simulink model "active_with_narx_and_can"  (R2024a)
settings: Solver=FixedStepAuto  StartTime=0.0  StopTime=40  FixedStep=0.005  RelTol=1e-3
undefined symbols (not defined in the file): A, B, C, canChannel, D, E, H, K1, K2, params, VehicleDataSingle
libraries: neural x41, j1939protocollib x5, vntj1939tllib x1, sldrtlib x1, simulink x1
(part 1 of 3)
settings Model: Creator=lwb  LastModifiedBy=lwb

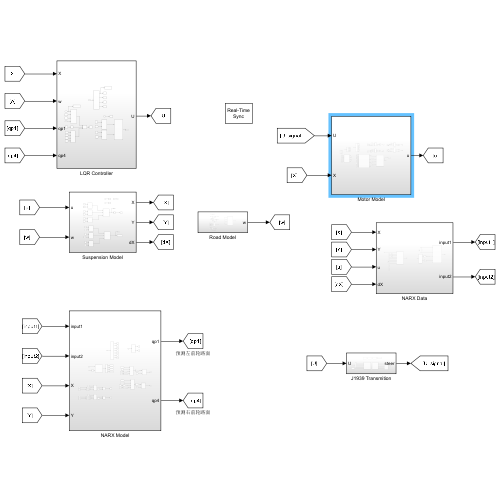
[thumbnail: Simulink's stored preview of the top-level diagram]
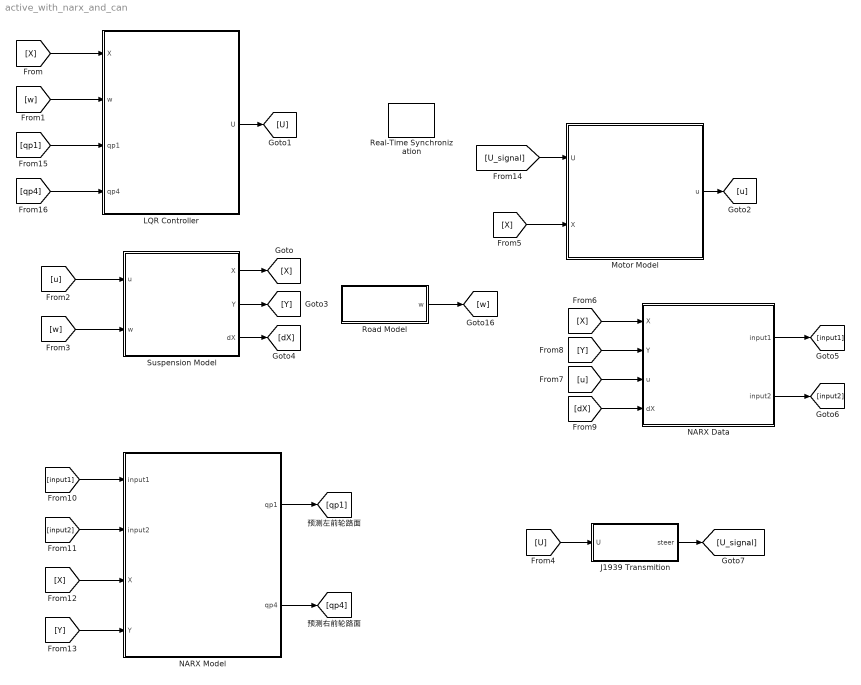
== system active_with_narx_and_can ==
  J1939 Transmition : Subsystem
  LQR Controller : Subsystem
  Motor Model : Subsystem
  NARX Data : Subsystem
  NARX Model : Subsystem
  Real-Time Synchronization : sldrtlib/Real-Time Synchronization  SampleTime=0.1  MaxMissedTicks=10  ShowMissedTicks=off  YieldWhenWaiting=off
  Road Model : Subsystem
  Suspension Model : Subsystem
  wires:
  [X] -> NARX Model/3(X)
  [input1] -> NARX Model/1(input1)
  LQR Controller/1(U) -> [U]
  NARX Data/1(input1) -> [input1]
  [u] -> NARX Data/3(u)
  [input2] -> NARX Model/2(input2)
  Road Model/1(w) -> [w]
  NARX Model/2(qp4) -> [qp4]
  NARX Model/1(qp1) -> [qp1]
  [w] -> LQR Controller/2(w)
  [qp4] -> LQR Controller/4(qp4)
  [u] -> Suspension Model/1(u)
  [Y] -> NARX Model/4(Y)
  [Y] -> NARX Data/2(Y)
  Motor Model/1(u) -> [u]
  NARX Data/2(input2) -> [input2]
  Suspension Model/3(dX) -> [dX]
  [X] -> LQR Controller/1(X)
  Suspension Model/2(Y) -> [Y]
  [dX] -> NARX Data/4(dX)
  [qp1] -> LQR Controller/3(qp1)
  Suspension Model/1(X) -> [X]
  [X] -> Motor Model/2(X)
  [X] -> NARX Data/1(X)
  [w] -> Suspension Model/2(w)
  J1939 Transmition/1(steer) -> [U_signal]
  [U] -> J1939 Transmition/1(U)
  [U_signal] -> Motor Model/1(U)

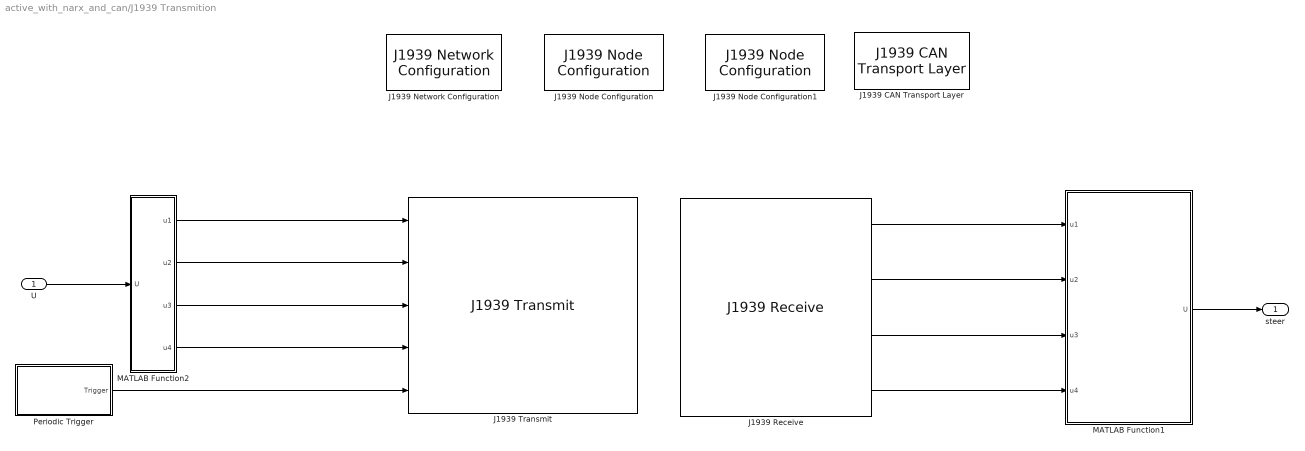
== system active_with_narx_and_can/J1939 Transmition ==
  U : Inport
  " Periodic Trigger" : Subsystem  mask(PeriodicTrigger){repetitionInterval=1}
      mask prompts: repetitionInterval "Repetition Interval (ms):"
      mask help: This block uses the wall-clock time to periodically output a trigger pulse
      mask init:
      | if repetitionInterval < 0
      |  error('xPCTarget:xpcblocks:j1939messagetrigger',...
      |        'Repetition Interval cannot be less than zero');
      | end
      mask Display: disp('Periodic Trigger \n Subsystem');
  J1939 CAN Transport Layer : vntj1939tllib/J1939 CAN Transport Layer  Priority=-2  DeviceMenu=MathWorks Virtual 1 (Channel 1)  ConfigName=Config1  ObjConstructor=canChannel('MathWorks', 'Virtual 1', 1)  Device=MathWorks Virtual 1 (Channel 1)  BusSpeedStr=250000  SampleTime=0.005
  J1939 Network Configuration : j1939protocollib/J1939 Network Configuration  Priority=-3  ConfigName=Config1  DbFile=C:\Users\lwb\Desktop\汽车电子大作业\model\J1939.dbc  PrevDbFile=C:\Users\lwb\Desktop\汽车电子大作业\model\J1939.dbc  enableAC=on
  J1939 Node Configuration : j1939protocollib/J1939 Node Configuration  Priority=-2  ConfigName=Config1  NodeID=Node1  NodeName=Node1  PrevNodeID=Custom  PrevConfig=Config  AllowAAC=off  NodeAddress=30  IndustryGroup=0  VehicleSystem=0  VehicleSystemInstance=0  FunctionID=22  FunctionInstance=0  ECUInstance=0  ManufacturerCode=0  IDNumber=0  SampleTime=0.005  OutputAddress=off  OutputACStatus=off
  J1939 Node Configuration1 : j1939protocollib/J1939 Node Configuration  Priority=-2  ConfigName=Config1  NodeID=Node2  NodeName=Node2  PrevNodeID=Custom  PrevConfig=Config  AllowAAC=off  NodeAddress=50  IndustryGroup=0  VehicleSystem=0  VehicleSystemInstance=0  FunctionID=8  FunctionInstance=0  ECUInstance=0  ManufacturerCode=0  IDNumber=0  SampleTime=0.005  OutputAddress=off  OutputACStatus=off
  J1939 Receive : j1939protocollib/J1939 Receive  Priority=-1  ConfigName=Config1  NodeName=Node2  PGList=VehicleDataSingle(40192)  PGName=VehicleDataSingle  MsgLength=8  SignalInfo=VehicleSignal1$0$16$1$1$1$0$1$0$-Inf$Inf$$0$#VehicleSignal2$16$16$1$1$1$0$1$0$-Inf$Inf$$0$#VehicleSignal3$32$16$1$1$1$0$1$0$-Inf$Inf$$0$#VehicleSignal4$48$16$1$1$1$0$1$0$-Inf$Inf$$0$#  NSignals=4  StartBits=str2num('[double(0);double(16);double(32);double(48)]')  SignalSizes=str2num('[double(16),double(16),double(16),double(16)]')  ByteOrders=str2num('[int32(1);int32(1);int32(1);int32(1)]')  DataTypes=str2num('[int32(1);int32(1);int32(1);int32(1)]')  MultiplexTypes=str2num('[int32(1);int32(1);int32(1);int32(1)]')  MultiplexValues=str2num('[double(0);double(0);double(0);double(0)]')  Factors=str2num('[double(1);double(1);double(1);double(1)]')  Offsets=str2num('[double(0);double(0);double(0);double(0)]')  Minimums=str2num('[double(-Inf);double(-Inf);double(-Inf);double(-Inf)]')  Maximums=str2num('[double(Inf);double(Inf);double(Inf);double(Inf)]')  Units=0  SPN=str2num('[double(0);double(0);double(0);double(0)]')  Comment=0  SrcAddrFilter=Allow all  SrcAddress=255  DestAddrFilter=1  outputNew=off  SampleTime=0.005  ApplyMinMax=off
  J1939 Transmit : j1939protocollib/J1939 Transmit  Priority=-1  ConfigName=Config1  NodeName=Node1  PGList=VehicleDataSingle(40192)  PGName=VehicleDataSingle  MsgLength=8  SignalInfo=VehicleSignal1$0$16$1$1$1$0$1$0$-Inf$Inf$$0$#VehicleSignal2$16$16$1$1$1$0$1$0$-Inf$Inf$$0$#VehicleSignal3$32$16$1$1$1$0$1$0$-Inf$Inf$$0$#VehicleSignal4$48$16$1$1$1$0$1$0$-Inf$Inf$$0$#  NSignals=4  StartBits=str2num('[double(0);double(16);double(32);double(48)]')  SignalSizes=str2num('[double(16),double(16),double(16),double(16)]')  ByteOrders=str2num('[int32(1);int32(1);int32(1);int32(1)]')  DataTypes=str2num('[int32(1);int32(1);int32(1);int32(1)]')  MultiplexTypes=str2num('[int32(1);int32(1);int32(1);int32(1)]')  MultiplexValues=str2num('[double(0);double(0);double(0);double(0)]')  Factors=str2num('[double(1);double(1);double(1);double(1)]')  Offsets=str2num('[double(0);double(0);double(0);double(0)]')  Minimums=str2num('[double(-Inf);double(-Inf);double(-Inf);double(-Inf)]')  Maximums=str2num('[double(Inf);double(Inf);double(Inf);double(Inf)]')  Units=0  SPN=str2num('[double(0);double(0);double(0);double(0)]')  Comment=0  PGPriority=6  DestAddrID=Node2  DestAddrName=50  TransmitPeriodically=on  MessagePeriod=0  SampleTime=-1  ApplyMinMax=off
  MATLAB Function1 : MATLAB Function  TreatAsAtomicUnit=on
  MATLAB Function2 : MATLAB Function  TreatAsAtomicUnit=on
  steer : Outport
  wires:
  U/1 -> MATLAB Function2/1(U)
  MATLAB Function1/1(U) -> steer/1
  " Periodic Trigger"/1(Trigger) -> J1939 Transmit/5
  MATLAB Function2/1(u1) -> J1939 Transmit/1
  MATLAB Function2/2(u2) -> J1939 Transmit/2
  MATLAB Function2/3(u3) -> J1939 Transmit/3
  MATLAB Function2/4(u4) -> J1939 Transmit/4
  J1939 Receive/1 -> MATLAB Function1/1(u1)
  J1939 Receive/2 -> MATLAB Function1/2(u2)
  J1939 Receive/3 -> MATLAB Function1/3(u3)
  J1939 Receive/4 -> MATLAB Function1/4(u4)

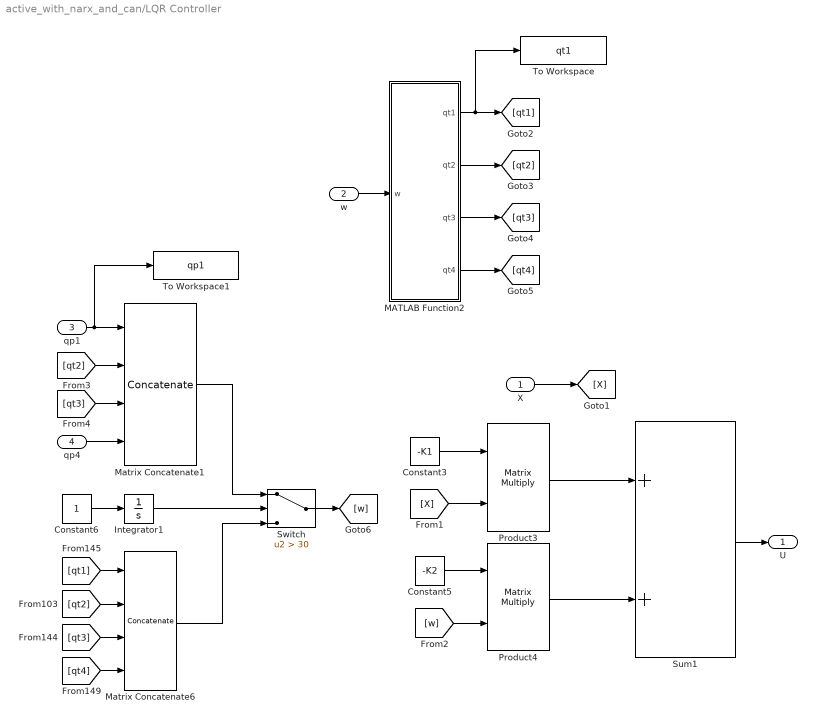
== system active_with_narx_and_can/LQR Controller ==
  X : Inport
  w : Inport  Port=2
  qp1 : Inport  Port=3
  qp4 : Inport  Port=4
  Constant3 : Constant  Value=-K1  VectorParams1D=off
  Constant5 : Constant  Value=-K2  VectorParams1D=off
  Constant6 : Constant
  Integrator1 : Integrator
  MATLAB Function2 : MATLAB Function  TreatAsAtomicUnit=on
  Matrix Concatenate1 : Concatenate  NumInputs=4  Mode=Multidimensional array
  Matrix Concatenate6 : Concatenate  NumInputs=4  Mode=Multidimensional array
  Product3 : Product  Multiplication=Matrix(*)
  Product4 : Product  Multiplication=Matrix(*)
  Sum1 : Sum
  Switch : Switch  Criteria=u2 > Threshold  Threshold=30  SaturateOnIntegerOverflow=off  InputSameDT=off
  To Workspace : ToWorkspace  VariableName=qt1  SaveFormat=Timeseries  SampleTime=-1
  To Workspace1 : ToWorkspace  VariableName=qp1  SaveFormat=Timeseries  SampleTime=-1
  U : Outport
  wires:
  [X] -> Product3/2
  Constant5/1 -> Product4/1
  Constant3/1 -> Product3/1
  Sum1/1 -> U/1
  Product3/1 -> Sum1/1
  Product4/1 -> Sum1/2
  [w] -> Product4/2
  X/1 -> [X]
  [qt2] -> Matrix Concatenate6/2
  [qt4] -> Matrix Concatenate6/4
  [qt3] -> Matrix Concatenate6/3
  Constant6/1 -> Integrator1/1
  [qt1] -> Matrix Concatenate6/1
  Integrator1/1 -> Switch/2
  w/1 -> MATLAB Function2/1(w)
  Switch/1 -> [w]
  qp1/1 -> To Workspace1/1, Matrix Concatenate1/1
  [qt2] -> Matrix Concatenate1/2
  qp4/1 -> Matrix Concatenate1/4
  [qt3] -> Matrix Concatenate1/3
  Matrix Concatenate1/1 -> Switch/1
  Matrix Concatenate6/1 -> Switch/3
  MATLAB Function2/3(qt3) -> [qt3]
  MATLAB Function2/2(qt2) -> [qt2]
  MATLAB Function2/4(qt4) -> [qt4]
  MATLAB Function2/1(qt1) -> To Workspace/1, [qt1]

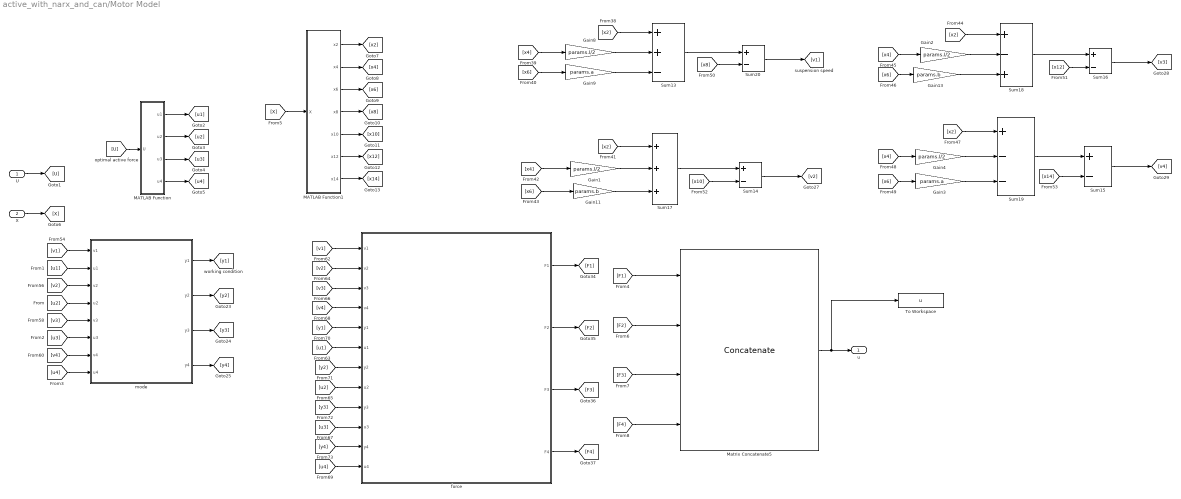
== system active_with_narx_and_can/Motor Model ==
  U : Inport
  X : Inport  Port=2
  Gain{1..2,4,8} (4 alike) : Gain  Gain=params.l/2
  Gain11 : Gain  Gain=params.b
  Gain13 : Gain  Gain=params.b
  Gain3 : Gain  Gain=params.a
  Gain9 : Gain  Gain=params.a
  MATLAB Function : MATLAB Function  TreatAsAtomicUnit=on
  MATLAB Function1 : MATLAB Function  TreatAsAtomicUnit=on
  Matrix Concatenate5 : Concatenate  NumInputs=4  Mode=Multidimensional array
  Sum13 : Sum  Inputs=++-
  Sum{14..16,20} (4 alike) : Sum  Inputs=+-
  Sum17 : Sum  Inputs=+++
  Sum18 : Sum  Inputs=+-+
  Sum19 : Sum  Inputs=+--
  To Workspace : ToWorkspace  VariableName=u  SaveFormat=Timeseries  SampleTime=-1
  force : Subsystem
  mode : Subsystem
  u : Outport
  wires:
  [y4] -> force/11(y4)
  [u1] -> force/6(u1)
  force/1(F1) -> [F1]
  force/2(F2) -> [F2]
  [v2] -> force/2(v2)
  mode/1(y1) -> [y1]
  [v3] -> force/3(v3)
  [u4] -> mode/8(u4)
  [u3] -> mode/6(u3)
  force/4(F4) -> [F4]
  [v4] -> force/4(v4)
  [y2] -> force/7(y2)
  [v3] -> mode/5(v3)
  mode/2(y2) -> [y2]
  [v4] -> mode/7(v4)
  [u4] -> force/12(u4)
  mode/4(y4) -> [y4]
  [u3] -> force/10(u3)
  mode/3(y3) -> [y3]
  [v2] -> mode/3(v2)
  [u2] -> force/8(u2)
  [v1] -> force/1(v1)
  [v1] -> mode/1(v1)
  [u2] -> mode/4(u2)
  [y3] -> force/9(y3)
  [u1] -> mode/2(u1)
  force/3(F3) -> [F3]
  [y1] -> force/5(y1)
  Sum19/1 -> Sum15/1
  [x14] -> Sum15/2
  Sum16/1 -> [v3]
  [x6] -> Gain13/1
  Gain8/1 -> Sum13/2
  [x2] -> Sum13/1
  Gain1/1 -> Sum17/2
  Sum20/1 -> [v1]
  [x2] -> Sum19/1
  [x4] -> Gain4/1
  [x6] -> Gain9/1
  [x2] -> Sum18/1
  Sum18/1 -> Sum16/1
  Gain9/1 -> Sum13/3
  Sum13/1 -> Sum20/1
  [x12] -> Sum16/2
  Sum15/1 -> [v4]
  Gain3/1 -> Sum19/3
  Gain2/1 -> Sum18/2
  [x4] -> Gain2/1
  [x4] -> Gain1/1
  Gain13/1 -> Sum18/3
  [x6] -> Gain11/1
  Sum17/1 -> Sum14/1
  Gain11/1 -> Sum17/3
  Gain4/1 -> Sum19/2
  [x10] -> Sum14/2
  [x2] -> Sum17/1
  [x4] -> Gain8/1
  Sum14/1 -> [v2]
  [x6] -> Gain3/1
  [x8] -> Sum20/2
  U/1 -> [U]
  [U] -> MATLAB Function/1(U)
  MATLAB Function/2(u2) -> [u2]
  MATLAB Function/3(u3) -> [u3]
  MATLAB Function/4(u4) -> [u4]
  MATLAB Function/1(u1) -> [u1]
  X/1 -> [X]
  [X] -> MATLAB Function1/1(X)
  MATLAB Function1/1(x2) -> [x2]
  MATLAB Function1/2(x4) -> [x4]
  MATLAB Function1/3(x6) -> [x6]
  MATLAB Function1/4(x8) -> [x8]
  MATLAB Function1/5(x10) -> [x10]
  MATLAB Function1/6(x12) -> [x12]
  MATLAB Function1/7(x14) -> [x14]
  [F1] -> Matrix Concatenate5/1
  [F3] -> Matrix Concatenate5/3
  [F4] -> Matrix Concatenate5/4
  [F2] -> Matrix Concatenate5/2
  Matrix Concatenate5/1 -> To Workspace/1, u/1

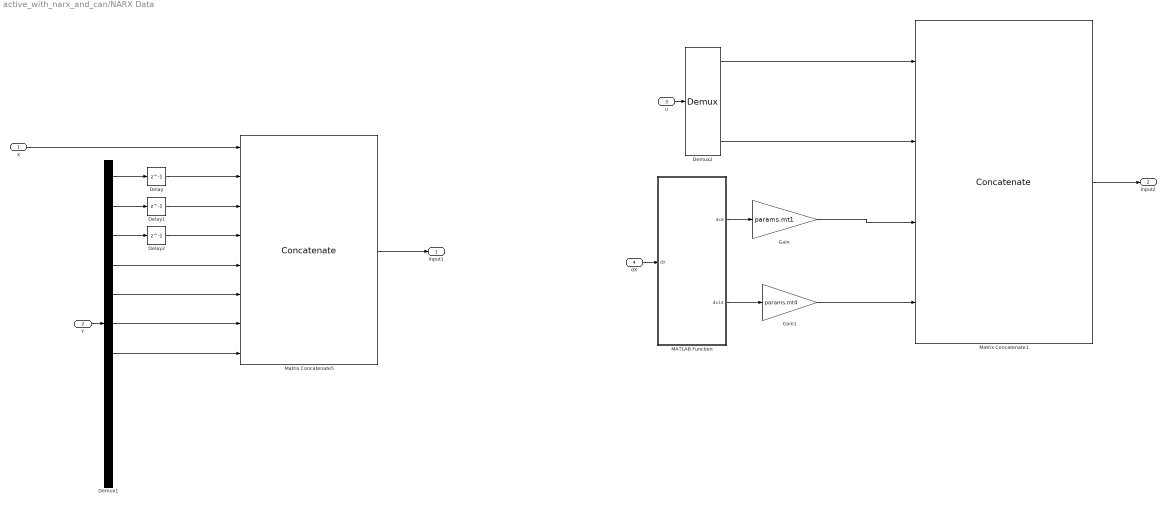
== system active_with_narx_and_can/NARX Data ==
  X : Inport
  Y : Inport  Port=2
  u : Inport  Port=3
  dX : Inport  Port=4
  Delay : Delay  DelayLength=1
  Delay1 : Delay  DelayLength=1
  Delay2 : Delay  DelayLength=1
  Demux1 : Demux  Outputs=11
  Demux2 : Demux
  Gain : Gain  Gain=params.mt1
  Gain1 : Gain  Gain=params.mt4
  MATLAB Function : MATLAB Function  TreatAsAtomicUnit=on
  Matrix Concatenate1 : Concatenate  NumInputs=4  Mode=Multidimensional array
  Matrix Concatenate5 : Concatenate  NumInputs=8  Mode=Multidimensional array
  input1 : Outport
  input2 : Outport  Port=2
  wires:
  Y/1 -> Demux1/1
  Demux1/1 -> Delay/1
  Demux1/2 -> Delay1/1
  Demux1/3 -> Delay2/1
  u/1 -> Demux2/1
  Demux2/1 -> Matrix Concatenate1/1
  Demux2/4 -> Matrix Concatenate1/2
  dX/1 -> MATLAB Function/1(dX)
  MATLAB Function/1(dx8) -> Gain/1
  MATLAB Function/2(dx14) -> Gain1/1
  Gain/1 -> Matrix Concatenate1/3
  Gain1/1 -> Matrix Concatenate1/4
  X/1 -> Matrix Concatenate5/1
  Delay/1 -> Matrix Concatenate5/2
  Delay1/1 -> Matrix Concatenate5/3
  Delay2/1 -> Matrix Concatenate5/4
  Demux1/4 -> Matrix Concatenate5/5
  Demux1/5 -> Matrix Concatenate5/6
  Demux1/6 -> Matrix Concatenate5/7
  Demux1/7 -> Matrix Concatenate5/8
  Matrix Concatenate5/1 -> input1/1
  Matrix Concatenate1/1 -> input2/1

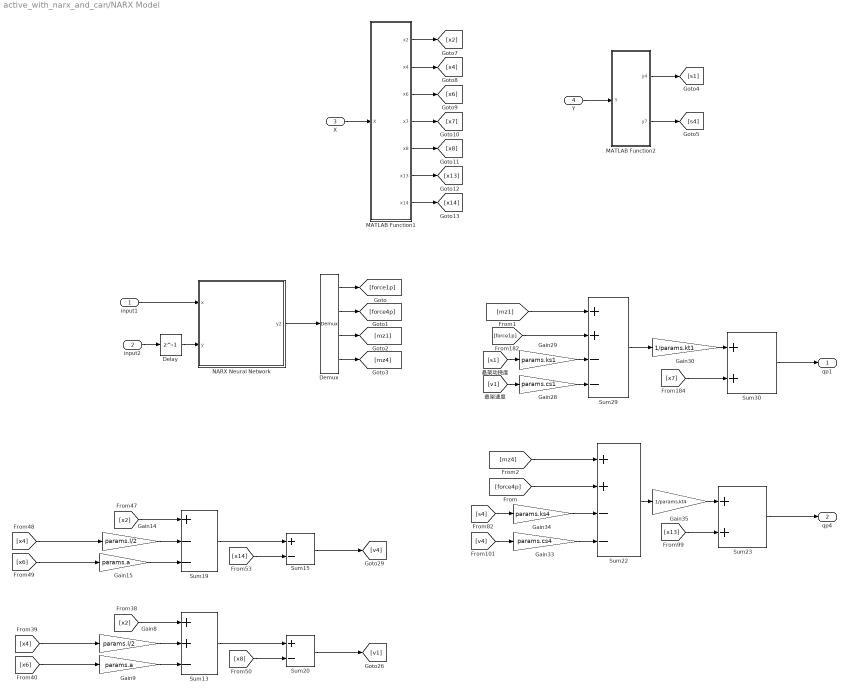
== system active_with_narx_and_can/NARX Model ==
  input1 : Inport
  input2 : Inport  Port=2
  X : Inport  Port=3
  Y : Inport  Port=4
  Delay : Delay  DelayLength=1
  Demux : Demux
  Gain14 : Gain  Gain=params.l/2
  Gain15 : Gain  Gain=params.a
  Gain28 : Gain  Gain=params.cs1
  Gain29 : Gain  Gain=params.ks1
  Gain30 : Gain  Gain=1/params.kt1
  Gain33 : Gain  Gain=params.cs4
  Gain34 : Gain  Gain=params.ks4
  Gain35 : Gain  Gain=1/params.kt4
  Gain8 : Gain  Gain=params.l/2
  Gain9 : Gain  Gain=params.a
  MATLAB Function1 : MATLAB Function  TreatAsAtomicUnit=on
  MATLAB Function2 : MATLAB Function  TreatAsAtomicUnit=on
  NARX Neural Network : Subsystem  mask{pi_input_1_delayed_1=[0;0;0;0;0;0;0;0;0;0;0;0;0;0;0;0;0;0;0;0;0], pi_input_1_delayed_2=[0;0;0;0;0;0;0;0;0;0;0;0;0;0;0;0;0;0;0;0;0], pi_input_2_delayed_1=[0;0;0;0], pi_input_2_delayed_2=[0;0;0;0]}
      mask prompts: pi_input_1_delayed_1 "Preprocessed initial input 1 state at timestep 0."; pi_input_1_delayed_2 "Preprocessed initial input 1 state at timestep -1."; pi_input_2_delayed_1 "Preprocessed initial input 2 state at timestep 0."; pi_input_2_delayed_2 "Preprocessed initial input 2 state at timestep -1."
      mask help: NARX Neural Network
      mask Display: e = 0.06;c1 = [120 150 230]/255;c2 = ([120 150 230]+0)/383;c3 = ([120 150 230]+128)/383;patch([0 1 1 0],[0 0 1 1],c1);patch([0 1 1 1-e 1-e 0+e],[0 0 1 1-e 0+e 0+e],c2);patch([0 0 1 1-e 0+e 0+e],[0 1 1 1-e 1-e 0+e],c3);plot([0 1 1 0 0],[0 0 1 1 0]);fprintf('NNET');port_label('input',1,' x');port_label('input',2,' y');port_label('output',1,'y2 ');
  Sum13 : Sum  Inputs=++-
  Sum15 : Sum  Inputs=+-
  Sum19 : Sum  Inputs=+--
  Sum20 : Sum  Inputs=+-
  Sum22 : Sum  Inputs=++--
  Sum23 : Sum
  Sum29 : Sum  Inputs=++--
  Sum30 : Sum
  qp1 : Outport
  qp4 : Outport  Port=2
  wires:
  Delay/1 -> NARX Neural Network/2(y)
  input2/1 -> Delay/1
  input1/1 -> NARX Neural Network/1(x)
  Gain30/1 -> Sum30/1
  Sum30/1 -> qp1/1
  Gain29/1 -> Sum29/3
  Gain33/1 -> Sum22/4
  [v1] -> Gain28/1
  [x13] -> Sum23/2
  [force4p] -> Sum22/2
  Gain35/1 -> Sum23/1
  [s1] -> Gain29/1
  Sum29/1 -> Gain30/1
  Sum22/1 -> Gain35/1
  Gain34/1 -> Sum22/3
  [s4] -> Gain34/1
  [force1p] -> Sum29/2
  Sum23/1 -> qp4/1
  [v4] -> Gain33/1
  [mz1] -> Sum29/1
  [mz4] -> Sum22/1
  [x7] -> Sum30/2
  Gain28/1 -> Sum29/4
  NARX Neural Network/1(y2) -> Demux/1
  Demux/1 -> [force1p]
  Demux/2 -> [force4p]
  Demux/3 -> [mz1]
  Demux/4 -> [mz4]
  [x2] -> Sum13/1
  [x4] -> Gain14/1
  [x8] -> Sum20/2
  Sum19/1 -> Sum15/1
  [x14] -> Sum15/2
  Sum13/1 -> Sum20/1
  Sum20/1 -> [v1]
  Gain14/1 -> Sum19/2
  [x6] -> Gain9/1
  Gain9/1 -> Sum13/3
  [x4] -> Gain8/1
  Sum15/1 -> [v4]
  Gain8/1 -> Sum13/2
  [x2] -> Sum19/1
  [x6] -> Gain15/1
  Gain15/1 -> Sum19/3
  MATLAB Function1/6(x13) -> [x13]
  MATLAB Function1/1(x2) -> [x2]
  MATLAB Function1/2(x4) -> [x4]
  MATLAB Function1/3(x6) -> [x6]
  X/1 -> MATLAB Function1/1(X)
  MATLAB Function1/7(x14) -> [x14]
  MATLAB Function1/4(x7) -> [x7]
  MATLAB Function1/5(x8) -> [x8]
  Y/1 -> MATLAB Function2/1(Y)
  MATLAB Function2/1(y4) -> [s1]
  MATLAB Function2/2(y7) -> [s4]

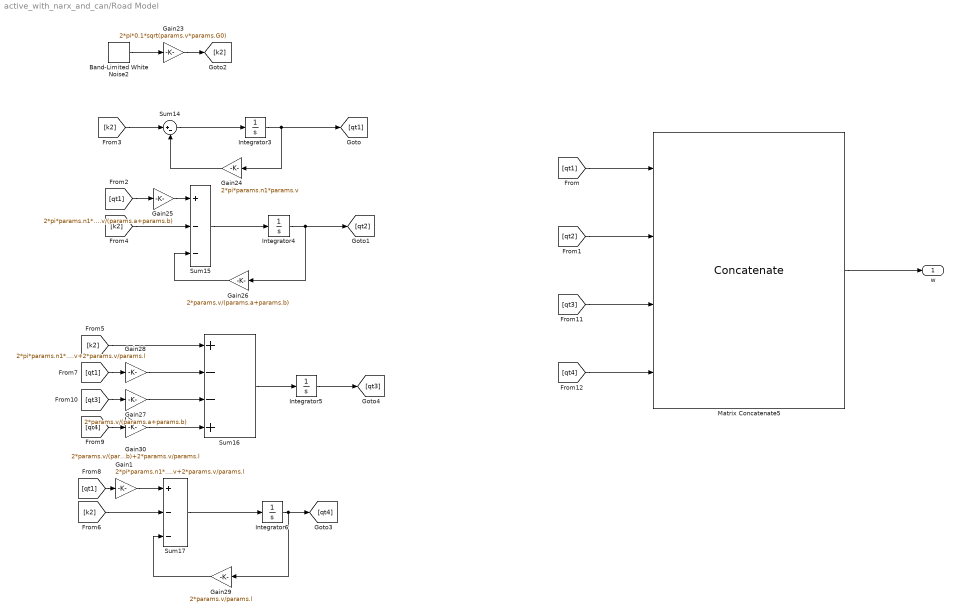
== system active_with_narx_and_can/Road Model ==
  Band-Limited White Noise2 : simulink/Sources/Band-Limited White Noise  Cov=[0.5]  Ts=1/10/params.v  seed=[23341]
  Gain1 : Gain  Gain=2*pi*params.n1*params.v+2*params.v/params.l
  Gain23 : Gain  Gain=2*pi*0.1*sqrt(params.v*params.G0)
  Gain24 : Gain  Gain=2*pi*params.n1*params.v
  Gain25 : Gain  Gain=2*pi*params.n1*params.v+2*params.v/(params.a+params.b)
  Gain26 : Gain  Gain=2*params.v/(params.a+params.b)
  Gain27 : Gain  Gain=2*params.v/(params.a+params.b)
  Gain28 : Gain  Gain=2*pi*params.n1*params.v+2*params.v/params.l
  Gain29 : Gain  Gain=2*params.v/params.l
  Gain30 : Gain  Gain=2*params.v/(params.a+params.b)+2*params.v/params.l
  Integrator{3..6} (4 alike) : Integrator
  Matrix Concatenate5 : Concatenate  NumInputs=4  Mode=Multidimensional array
  Sum14 : Sum  Inputs=|+-
  Sum15 : Sum  Inputs=+--
  Sum16 : Sum  Inputs=+--+
  Sum17 : Sum  Inputs=+--
  w : Outport
  wires:
  Gain25/1 -> Sum15/1
  Gain27/1 -> Sum16/3
  Gain26/1 -> Sum15/3
  Gain24/1 -> Sum14/2
  Integrator5/1 -> [qt3]
  Integrator3/1 -> Gain24/1, [qt1]
  Matrix Concatenate5/1 -> w/1
  Sum14/1 -> Integrator3/1
  Integrator4/1 -> Gain26/1, [qt2]
  Integrator6/1 -> Gain29/1, [qt4]
  Gain28/1 -> Sum16/2
  Gain29/1 -> Sum17/3
  Sum16/1 -> Integrator5/1
  Sum15/1 -> Integrator4/1
  Gain30/1 -> Sum16/4
  Sum17/1 -> Integrator6/1
  [k2] -> Sum14/1
  Band-Limited White Noise2/1 -> Gain23/1
  Gain23/1 -> [k2]
  [k2] -> Sum15/2
  [k2] -> Sum16/1
  [k2] -> Sum17/2
  [qt1] -> Gain25/1
  [qt1] -> Gain28/1
  [qt1] -> Gain1/1
  Gain1/1 -> Sum17/1
  [qt3] -> Gain27/1
  [qt4] -> Gain30/1
  [qt3] -> Matrix Concatenate5/3
  [qt4] -> Matrix Concatenate5/4
  [qt1] -> Matrix Concatenate5/1
  [qt2] -> Matrix Concatenate5/2

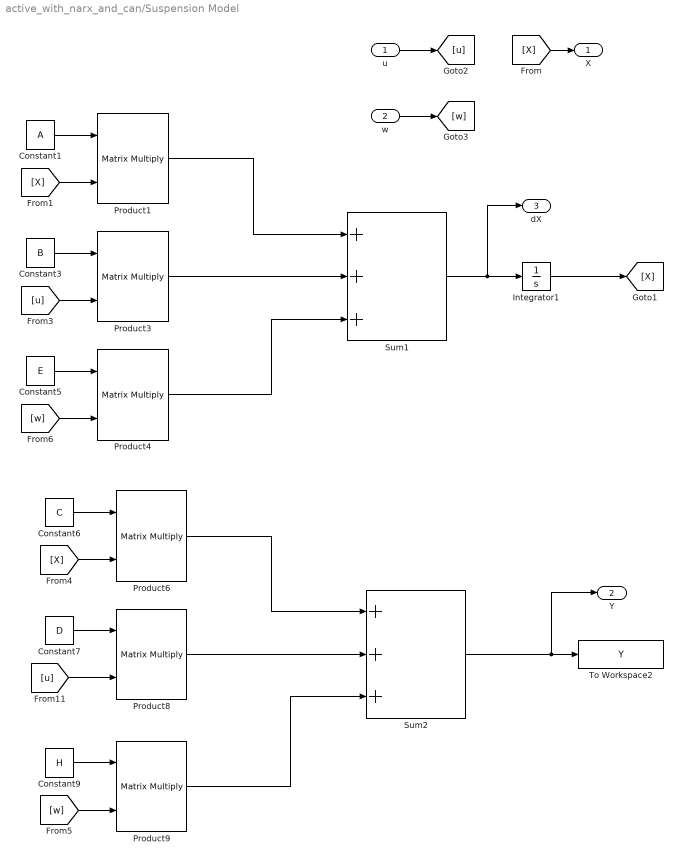
== system active_with_narx_and_can/Suspension Model ==
  u : Inport
  w : Inport  Port=2
  Constant1 : Constant  Value=A  VectorParams1D=off
  Constant3 : Constant  Value=B  VectorParams1D=off
  Constant5 : Constant  Value=E  VectorParams1D=off
  Constant6 : Constant  Value=C  VectorParams1D=off
  Constant7 : Constant  Value=D  VectorParams1D=off
  Constant9 : Constant  Value=H  VectorParams1D=off
  Integrator1 : Integrator
  Product{1,3..4,6,8..9} (6 alike) : Product  Multiplication=Matrix(*)
  Sum1 : Sum  Inputs=+++
  Sum2 : Sum  Inputs=+++
  To Workspace2 : ToWorkspace  VariableName=Y  SaveFormat=Timeseries  SampleTime=-1
  X : Outport
  Y : Outport  Port=2
  dX : Outport  Port=3
  wires:
  Constant3/1 -> Product3/1
  [u] -> Product8/2
  Product4/1 -> Sum1/3
  [u] -> Product3/2
  Product1/1 -> Sum1/1
  Constant1/1 -> Product1/1
  Product6/1 -> Sum2/1
  Sum1/1 -> dX/1, Integrator1/1
  Product9/1 -> Sum2/3
  [X] -> Product1/2
  Product8/1 -> Sum2/2
  Constant7/1 -> Product8/1
  [w] -> Product9/2
  Constant9/1 -> Product9/1
  Constant6/1 -> Product6/1
  Sum2/1 -> Y/1, To Workspace2/1
  Product3/1 -> Sum1/2
  [X] -> Product6/2
  [w] -> Product4/2
  Constant5/1 -> Product4/1
  u/1 -> [u]
  w/1 -> [w]
  Integrator1/1 -> [X]
  [X] -> X/1

== system active_with_narx_and_can/J1939 Transmition/ Periodic Trigger ==
  Relational Operator : RelationalOperator  OutDataTypeStr=boolean  InputSameDT=off
  Repetition Interval : Constant  Value=repetitionInterval
  Timer : Subsystem
  Unit Delay : UnitDelay  InitialCondition=1  SampleTime=-1  HasFrameUpgradeWarning=on
  Trigger : Outport  OutputWhenDisabled=reset  InitialOutput=0  VectorParamsAs1DForOutWhenUnconnected=off
  wires:
  Timer/1(Timer Value (ms)) -> Relational Operator/1
  Repetition Interval/1 -> Relational Operator/2
  Unit Delay/1 -> Timer/1(Reset)
  Relational Operator/1 -> Trigger/1, Unit Delay/1  "Trigger Pulse"

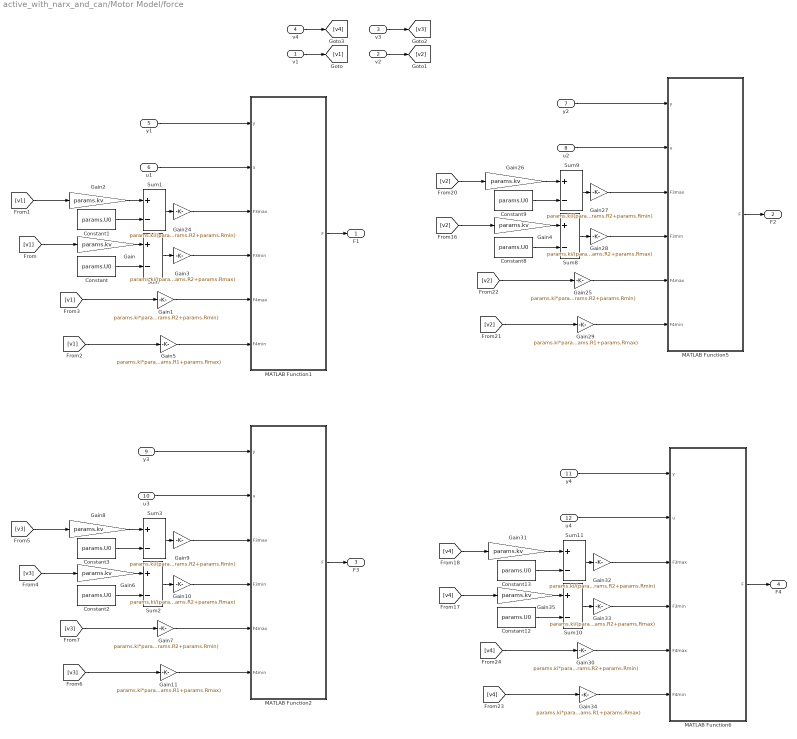
== system active_with_narx_and_can/Motor Model/force ==
  v1 : Inport
  v2 : Inport  Port=2
  v3 : Inport  Port=3
  v4 : Inport  Port=4
  y1 : Inport  Port=5
  u1 : Inport  Port=6
  y2 : Inport  Port=7
  u2 : Inport  Port=8
  y3 : Inport  Port=9
  u3 : Inport  Port=10
  y4 : Inport  Port=11
  u4 : Inport  Port=12
  Constant{,1..3,8..9,12..13} (8 alike) : Constant  Value=params.U0
  Gain{,2,4,6,8,26,31,35} (8 alike) : Gain  Gain=params.kv
  Gain{1,7,25,30} (4 alike) : Gain  Gain=params.ki*params.kv/(params.R2+params.Rmin)
  Gain{3,10,28,33} (4 alike) : Gain  Gain=params.ki/(params.R1+params.R2+params.Rmax)
  Gain{5,11,29,34} (4 alike) : Gain  Gain=params.ki*params.kv/(params.R1+params.Rmax)
  Gain{9,24,27,32} (4 alike) : Gain  Gain=params.ki/(params.R1+params.R2+params.Rmin)
  MATLAB Function1 : MATLAB Function  TreatAsAtomicUnit=on
  MATLAB Function2 : MATLAB Function  TreatAsAtomicUnit=on
  MATLAB Function5 : MATLAB Function  TreatAsAtomicUnit=on
  MATLAB Function6 : MATLAB Function  TreatAsAtomicUnit=on
  Sum{,1..3,8..11} (8 alike) : Sum  Inputs=+-
  F1 : Outport
  F2 : Outport  Port=2
  F3 : Outport  Port=3
  F4 : Outport  Port=4
  wires:
  v4/1 -> [v4]
  Gain3/1 -> MATLAB Function1/4(F3min)
  Gain1/1 -> MATLAB Function1/5(F4max)
  v3/1 -> [v3]
  v2/1 -> [v2]
  [v1] -> Gain1/1
  Gain5/1 -> MATLAB Function1/6(F4min)
  Gain24/1 -> MATLAB Function1/3(F3max)
  [v1] -> Gain/1
  v1/1 -> [v1]
  Constant1/1 -> Sum1/2
  Sum1/1 -> Gain24/1
  Sum/1 -> Gain3/1
  Constant/1 -> Sum/2
  Gain/1 -> Sum/1
  y1/1 -> MATLAB Function1/1(y)
  u1/1 -> MATLAB Function1/2(u)
  [v1] -> Gain2/1
  Gain2/1 -> Sum1/1
  [v1] -> Gain5/1
  MATLAB Function1/1(F) -> F1/1
  MATLAB Function5/1(F) -> F2/1
  [v2] -> Gain29/1
  Gain26/1 -> Sum9/1
  [v2] -> Gain26/1
  u2/1 -> MATLAB Function5/2(u)
  y2/1 -> MATLAB Function5/1(y)
  Gain4/1 -> Sum8/1
  Constant8/1 -> Sum8/2
  Sum8/1 -> Gain28/1
  Sum9/1 -> Gain27/1
  Constant9/1 -> Sum9/2
  [v2] -> Gain4/1
  Gain27/1 -> MATLAB Function5/3(F3max)
  Gain29/1 -> MATLAB Function5/6(F4min)
  [v2] -> Gain25/1
  Gain25/1 -> MATLAB Function5/5(F4max)
  Gain28/1 -> MATLAB Function5/4(F3min)
  MATLAB Function2/1(F) -> F3/1
  [v3] -> Gain11/1
  Gain8/1 -> Sum3/1
  [v3] -> Gain8/1
  u3/1 -> MATLAB Function2/2(u)
  y3/1 -> MATLAB Function2/1(y)
  Gain6/1 -> Sum2/1
  Constant2/1 -> Sum2/2
  Sum2/1 -> Gain10/1
  Sum3/1 -> Gain9/1
  Constant3/1 -> Sum3/2
  [v3] -> Gain6/1
  Gain9/1 -> MATLAB Function2/3(F3max)
  Gain11/1 -> MATLAB Function2/6(F4min)
  [v3] -> Gain7/1
  Gain7/1 -> MATLAB Function2/5(F4max)
  Gain10/1 -> MATLAB Function2/4(F3min)
  Gain33/1 -> MATLAB Function6/4(F3min)
  Gain30/1 -> MATLAB Function6/5(F4max)
  [v4] -> Gain30/1
  Gain34/1 -> MATLAB Function6/6(F4min)
  Gain32/1 -> MATLAB Function6/3(F3max)
  [v4] -> Gain35/1
  Constant13/1 -> Sum11/2
  Sum11/1 -> Gain32/1
  Sum10/1 -> Gain33/1
  Constant12/1 -> Sum10/2
  Gain35/1 -> Sum10/1
  y4/1 -> MATLAB Function6/1(y)
  u4/1 -> MATLAB Function6/2(u)
  [v4] -> Gain31/1
  Gain31/1 -> Sum11/1
  [v4] -> Gain34/1
  MATLAB Function6/1(F) -> F4/1

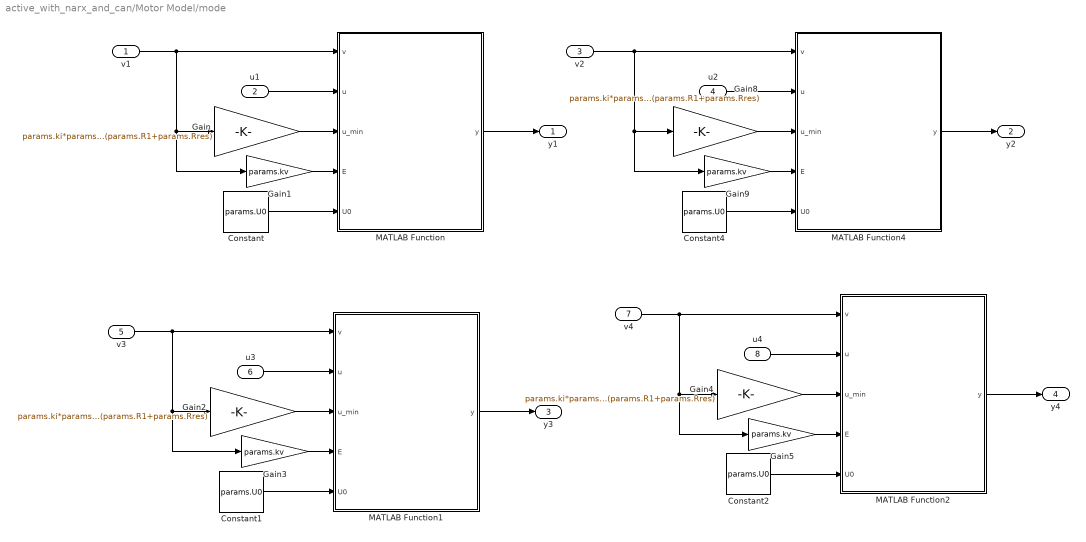
== system active_with_narx_and_can/Motor Model/mode ==
  v1 : Inport
  u1 : Inport  Port=2
  v2 : Inport  Port=3
  u2 : Inport  Port=4
  v3 : Inport  Port=5
  u3 : Inport  Port=6
  v4 : Inport  Port=7
  u4 : Inport  Port=8
  Constant{,1..2,4} (4 alike) : Constant  Value=params.U0
  Gain{,2,4,8} (4 alike) : Gain  Gain=params.ki*params.kv/(params.R1+params.Rres)
  Gain{1,3,5,9} (4 alike) : Gain  Gain=params.kv
  MATLAB Function : MATLAB Function  TreatAsAtomicUnit=on
  MATLAB Function1 : MATLAB Function  TreatAsAtomicUnit=on
  MATLAB Function2 : MATLAB Function  TreatAsAtomicUnit=on
  MATLAB Function4 : MATLAB Function  TreatAsAtomicUnit=on
  y1 : Outport
  y2 : Outport  Port=2
  y3 : Outport  Port=3
  y4 : Outport  Port=4
  wires:
  v1/1 -> MATLAB Function/1(v), Gain1/1, Gain/1
  u1/1 -> MATLAB Function/2(u)
  Gain/1 -> MATLAB Function/3(u_min)
  Gain1/1 -> MATLAB Function/4(E)
  Constant/1 -> MATLAB Function/5(U0)
  MATLAB Function/1(y) -> y1/1
  MATLAB Function4/1(y) -> y2/1
  Constant4/1 -> MATLAB Function4/5(U0)
  Gain9/1 -> MATLAB Function4/4(E)
  Gain8/1 -> MATLAB Function4/3(u_min)
  u2/1 -> MATLAB Function4/2(u)
  v2/1 -> Gain8/1, Gain9/1, MATLAB Function4/1(v)
  MATLAB Function1/1(y) -> y3/1
  Constant1/1 -> MATLAB Function1/5(U0)
  Gain3/1 -> MATLAB Function1/4(E)
  Gain2/1 -> MATLAB Function1/3(u_min)
  u3/1 -> MATLAB Function1/2(u)
  v3/1 -> Gain2/1, Gain3/1, MATLAB Function1/1(v)
  v4/1 -> MATLAB Function2/1(v), Gain5/1, Gain4/1
  u4/1 -> MATLAB Function2/2(u)
  Gain4/1 -> MATLAB Function2/3(u_min)
  Gain5/1 -> MATLAB Function2/4(E)
  Constant2/1 -> MATLAB Function2/5(U0)
  MATLAB Function2/1(y) -> y4/1

== system active_with_narx_and_can/NARX Model/NARX Neural Network ==
  x : Inport  PortDimensions=21
      mask Display: e = 0.06;c1 = [120 230 180]/255;c2 = ([120 230 180]+0)/(256+128);c3 = ([120 230 180]+128)/(256+128);patch([0 1 1 0],[0 0 1 1],c1);patch([0 1 1 1-e 1-e 0+e],[0 0 1 1-e 0+e 0+e],c2);patch([0 0 1 1-e 0+e 0+e],[0 1 1 1-e 1-e 0+e],c3);plot([0 1 1 0 0],[0 0 1 1 0]);
  y : Inport  Port=2  PortDimensions=4
      mask Display: e = 0.06;c1 = [120 230 180]/255;c2 = ([120 230 180]+0)/(256+128);c3 = ([120 230 180]+128)/(256+128);patch([0 1 1 0],[0 0 1 1],c1);patch([0 1 1 1-e 1-e 0+e],[0 0 1 1-e 0+e 0+e],c2);patch([0 0 1 1-e 0+e 0+e],[0 1 1 1-e 1-e 0+e],c3);plot([0 1 1 0 0],[0 0 1 1 0]);
  Layer 1 : Subsystem
      mask Display: e = 0.06;c1 = [120 150 230]/255;c2 = ([120 150 230]+0)/383;c3 = ([120 150 230]+128)/383;patch([0 1 1 0],[0 0 1 1],c1);patch([0 1 1 1-e 1-e 0+e],[0 0 1 1-e 0+e 0+e],c2);patch([0 0 1 1-e 0+e 0+e],[0 1 1 1-e 1-e 0+e],c3);plot([0 1 1 0 0],[0 0 1 1 0]);
  Layer 2 : Subsystem
      mask Display: e = 0.06;c1 = [120 150 230]/255;c2 = ([120 150 230]+0)/383;c3 = ([120 150 230]+128)/383;patch([0 1 1 0],[0 0 1 1],c1);patch([0 1 1 1-e 1-e 0+e],[0 0 1 1-e 0+e 0+e],c2);patch([0 0 1 1-e 0+e 0+e],[0 1 1 1-e 1-e 0+e],c3);plot([0 1 1 0 0],[0 0 1 1 0]);
  Process Input 1 : Subsystem
      mask Display: e = 0.06;c1 = [120 150 230]/255;c2 = ([120 150 230]+0)/383;c3 = ([120 150 230]+128)/383;patch([0 1 1 0],[0 0 1 1],c1);patch([0 1 1 1-e 1-e 0+e],[0 0 1 1-e 0+e 0+e],c2);patch([0 0 1 1-e 0+e 0+e],[0 1 1 1-e 1-e 0+e],c3);plot([0 1 1 0 0],[0 0 1 1 0]);
  Process Input 2 : Subsystem
      mask Display: e = 0.06;c1 = [120 150 230]/255;c2 = ([120 150 230]+0)/383;c3 = ([120 150 230]+128)/383;patch([0 1 1 0],[0 0 1 1],c1);patch([0 1 1 1-e 1-e 0+e],[0 0 1 1-e 0+e 0+e],c2);patch([0 0 1 1-e 0+e 0+e],[0 1 1 1-e 1-e 0+e],c3);plot([0 1 1 0 0],[0 0 1 1 0]);
  Process Output 1 : Subsystem
      mask Display: e = 0.06;c1 = [120 150 230]/255;c2 = ([120 150 230]+0)/383;c3 = ([120 150 230]+128)/383;patch([0 1 1 0],[0 0 1 1],c1);patch([0 1 1 1-e 1-e 0+e],[0 0 1 1-e 0+e 0+e],c2);patch([0 0 1 1-e 0+e 0+e],[0 1 1 1-e 1-e 0+e],c3);plot([0 1 1 0 0],[0 0 1 1 0]);
  y2 : Outport  InitialOutput=[0;0;0;0]
      mask Display: e = 0.06;c1 = [120 230 180]/255;c2 = ([120 230 180]+0)/(256+128);c3 = ([120 230 180]+128)/(256+128);patch([0 1 1 0],[0 0 1 1],c1);patch([0 1 1 1-e 1-e 0+e],[0 0 1 1-e 0+e 0+e],c2);patch([0 0 1 1-e 0+e 0+e],[0 1 1 1-e 1-e 0+e],c3);plot([0 1 1 0 0],[0 0 1 1 0]);
  wires:
  x/1 -> Process Input 1/1(x)
  y/1 -> Process Input 2/1(x)
  Process Output 1/1(y) -> y2/1
  Process Input 1/1(p) -> Layer 1/1("p{1}")
  Process Input 2/1(p) -> Layer 1/2("p{2}")
  Layer 1/1("a{1}") -> [feedback1]
  [feedback1] -> Layer 2/1("a{1} ")
  Layer 2/1("a{2}") -> Process Output 1/1(a)

== system active_with_narx_and_can/J1939 Transmition/ Periodic Trigger/Timer ==
  Reset : Inport
  Constant : Constant  Value=eps
  Gain : Gain  Gain=1e3
  Logical Operator : Logic  Operator=NOT  AllPortsSameDT=off  OutDataTypeStr=boolean
  MATLAB Function : MATLAB Function  TreatAsAtomicUnit=on
  Sum : Sum  Inputs=-+
  Sum1 : Sum  Inputs=|++
  Switch : Switch  Criteria=u2 > Threshold  ZeroCross=off  SaturateOnIntegerOverflow=off  InputSameDT=off
  Unit Delay : UnitDelay  SampleTime=-1  HasFrameUpgradeWarning=on
  Unit Delay1 : UnitDelay  SampleTime=-1  HasFrameUpgradeWarning=on
  Timer Value (ms) : Outport  VectorParamsAs1DForOutWhenUnconnected=off
  wires:
  Gain/1 -> Timer Value (ms)/1
  Constant/1 -> Sum1/2
  Sum1/1 -> Gain/1
  Sum/1 -> Sum1/1
  Logical Operator/1 -> Switch/2
  MATLAB Function/1(y) -> Sum/2, Unit Delay1/1
  Unit Delay1/1 -> Switch/3
  Switch/1 -> Unit Delay/1, Sum/1
  Unit Delay/1 -> Switch/1
  Reset/1 -> Logical Operator/1

== system active_with_narx_and_can/NARX Model/NARX Neural Network/Layer 1 ==
  "p{1}" : Inport  PortDimensions=21
      mask Display: e = 0.06;c1 = [120 230 180]/255;c2 = ([120 230 180]+0)/(256+128);c3 = ([120 230 180]+128)/(256+128);patch([0 1 1 0],[0 0 1 1],c1);patch([0 1 1 1-e 1-e 0+e],[0 0 1 1-e 0+e 0+e],c2);patch([0 0 1 1-e 0+e 0+e],[0 1 1 1-e 1-e 0+e],c3);plot([0 1 1 0 0],[0 0 1 1 0]);
  "p{2}" : Inport  Port=2  PortDimensions=4
      mask Display: e = 0.06;c1 = [120 230 180]/255;c2 = ([120 230 180]+0)/(256+128);c3 = ([120 230 180]+128)/(256+128);patch([0 1 1 0],[0 0 1 1],c1);patch([0 1 1 1-e 1-e 0+e],[0 0 1 1-e 0+e 0+e],c2);patch([0 0 1 1-e 0+e 0+e],[0 1 1 1-e 1-e 0+e],c3);plot([0 1 1 0 0],[0 0 1 1 0]);
  Delays 1 : Subsystem
      mask Display: e = 0.06;c1 = [120 150 230]/255;c2 = ([120 150 230]+0)/383;c3 = ([120 150 230]+128)/383;patch([0 1 1 0],[0 0 1 1],c1);patch([0 1 1 1-e 1-e 0+e],[0 0 1 1-e 0+e 0+e],c2);patch([0 0 1 1-e 0+e 0+e],[0 1 1 1-e 1-e 0+e],c3);plot([0 1 1 0 0],[0 0 1 1 0]);disp('1-2');
  Delays 2 : Subsystem
      mask Display: e = 0.06;c1 = [120 150 230]/255;c2 = ([120 150 230]+0)/383;c3 = ([120 150 230]+128)/383;patch([0 1 1 0],[0 0 1 1],c1);patch([0 1 1 1-e 1-e 0+e],[0 0 1 1-e 0+e 0+e],c2);patch([0 0 1 1-e 0+e 0+e],[0 1 1 1-e 1-e 0+e],c3);plot([0 1 1 0 0],[0 0 1 1 0]);disp('1-2');
  "IW{1,1}" : Subsystem
      mask Display: e = 0.06;c1 = [120 150 230]/255;c2 = ([120 150 230]+0)/383;c3 = ([120 150 230]+128)/383;patch([0 1 1 0],[0 0 1 1],c1);patch([0 1 1 1-e 1-e 0+e],[0 0 1 1-e 0+e 0+e],c2);patch([0 0 1 1-e 0+e 0+e],[0 1 1 1-e 1-e 0+e],c3);plot([0 1 1 0 0],[0 0 1 1 0]);disp('W');
  "IW{1,2}" : Subsystem
      mask Display: e = 0.06;c1 = [120 150 230]/255;c2 = ([120 150 230]+0)/383;c3 = ([120 150 230]+128)/383;patch([0 1 1 0],[0 0 1 1],c1);patch([0 1 1 1-e 1-e 0+e],[0 0 1 1-e 0+e 0+e],c2);patch([0 0 1 1-e 0+e 0+e],[0 1 1 1-e 1-e 0+e],c3);plot([0 1 1 0 0],[0 0 1 1 0]);disp('W');
  "b{1}" : Constant  Value=[0.0362569717583896278245703115317155607044696807861328125;0.0267812047532714238295969977343702339567244052886962890625;-0.05313158255440302013550279980336199514567852020263671875;0.06369486160035824073855081906003761105239391326904296875;-0.386033597652299220737148743864963762462139129638671875;-0.34734839861144950479143744814791716635227203369140625;0.303550966296317004111671167265740223228931427001953125;0.4908053901393925055884892572066746652126312255859375;-0.68425446523709909651955740628181956708431243896484375;-0.1997581177343854264005784671098808757960796356201171875;0.05912996606181032677174158607158460654318332672119140625;-0.1657775452885270339731249578107963316142559051513671875;-0.233112932035969222521742949538747780025005340576171875;-0.2124324383006564176401553822870482690632343292236328125;0.471050002511267329463606756689841859042644500732421875;-0.6754084233547832383237619069404900074005126953125]
      mask Display: e = 0.06;c1 = [120 150 230]/255;c2 = ([120 150 230]+0)/383;c3 = ([120 150 230]+128)/383;patch([0 1 1 0],[0 0 1 1],c1);patch([0 1 1 1-e 1-e 0+e],[0 0 1 1-e 0+e 0+e],c2);patch([0 0 1 1-e 0+e 0+e],[0 1 1 1-e 1-e 0+e],c3);plot([0 1 1 0 0],[0 0 1 1 0]);disp('b');
  netsum : Sum  Inputs=3  InputSameDT=on  SaturateOnIntegerOverflow=on  OutDataTypeStr=Inherit: Same as first input
      mask Display: e = 0.06;c1 = [120 150 230]/255;c2 = ([120 150 230]+0)/383;c3 = ([120 150 230]+128)/383;patch([0 1 1 0],[0 0 1 1],c1);patch([0 1 1 1-e 1-e 0+e],[0 0 1 1-e 0+e 0+e],c2);patch([0 0 1 1-e 0+e 0+e],[0 1 1 1-e 1-e 0+e],c3);plot([0 1 1 0 0],[0 0 1 1 0]);disp('+');
  tansig : neural/Transfer Functions/tansig
  "a{1}" : Outport  InitialOutput=[0;0;0;0;0;0;0;0;0;0;0;0;0;0;0;0]
      mask Display: e = 0.06;c1 = [120 230 180]/255;c2 = ([120 230 180]+0)/(256+128);c3 = ([120 230 180]+128)/(256+128);patch([0 1 1 0],[0 0 1 1],c1);patch([0 1 1 1-e 1-e 0+e],[0 0 1 1-e 0+e 0+e],c2);patch([0 0 1 1-e 0+e 0+e],[0 1 1 1-e 1-e 0+e],c3);plot([0 1 1 0 0],[0 0 1 1 0]);
  wires:
  "p{1}"/1 -> Delays 1/1("p{1}")
  Delays 1/1("pd{1,1}") -> "IW{1,1}"/1("pd{1,1}")
  "IW{1,1}"/1("iz{1,1}") -> netsum/1
  "p{2}"/1 -> Delays 2/1("p{1}")
  Delays 2/1("pd{1,2}") -> "IW{1,2}"/1("pd{1,2}")
  "IW{1,2}"/1("iz{1,2}") -> netsum/2
  "b{1}"/1 -> netsum/3
  netsum/1 -> tansig/1
  tansig/1 -> "a{1}"/1

== system active_with_narx_and_can/NARX Model/NARX Neural Network/Layer 2 ==
  "a{1} " : Inport  PortDimensions=16
      mask Display: e = 0.06;c1 = [120 230 180]/255;c2 = ([120 230 180]+0)/(256+128);c3 = ([120 230 180]+128)/(256+128);patch([0 1 1 0],[0 0 1 1],c1);patch([0 1 1 1-e 1-e 0+e],[0 0 1 1-e 0+e 0+e],c2);patch([0 0 1 1-e 0+e 0+e],[0 1 1 1-e 1-e 0+e],c3);plot([0 1 1 0 0],[0 0 1 1 0]);
  Delays 1 : Subsystem
      mask Display: e = 0.06;c1 = [120 150 230]/255;c2 = ([120 150 230]+0)/383;c3 = ([120 150 230]+128)/383;patch([0 1 1 0],[0 0 1 1],c1);patch([0 1 1 1-e 1-e 0+e],[0 0 1 1-e 0+e 0+e],c2);patch([0 0 1 1-e 0+e 0+e],[0 1 1 1-e 1-e 0+e],c3);plot([0 1 1 0 0],[0 0 1 1 0]);disp('0');
  "LW{2,1}" : Subsystem
      mask Display: e = 0.06;c1 = [120 150 230]/255;c2 = ([120 150 230]+0)/383;c3 = ([120 150 230]+128)/383;patch([0 1 1 0],[0 0 1 1],c1);patch([0 1 1 1-e 1-e 0+e],[0 0 1 1-e 0+e 0+e],c2);patch([0 0 1 1-e 0+e 0+e],[0 1 1 1-e 1-e 0+e],c3);plot([0 1 1 0 0],[0 0 1 1 0]);disp('W');
  "b{2}" : Constant  Value=[0.1702662348160869643098891401677974499762058258056640625;0.1551065403463531000571862250581034459173679351806640625;-0.33225578068803274245368584161042235791683197021484375;0.489838588433543942191050746259861625730991363525390625]
      mask Display: e = 0.06;c1 = [120 150 230]/255;c2 = ([120 150 230]+0)/383;c3 = ([120 150 230]+128)/383;patch([0 1 1 0],[0 0 1 1],c1);patch([0 1 1 1-e 1-e 0+e],[0 0 1 1-e 0+e 0+e],c2);patch([0 0 1 1-e 0+e 0+e],[0 1 1 1-e 1-e 0+e],c3);plot([0 1 1 0 0],[0 0 1 1 0]);disp('b');
  netsum : Sum  Inputs=2  InputSameDT=on  SaturateOnIntegerOverflow=on  OutDataTypeStr=Inherit: Same as first input
      mask Display: e = 0.06;c1 = [120 150 230]/255;c2 = ([120 150 230]+0)/383;c3 = ([120 150 230]+128)/383;patch([0 1 1 0],[0 0 1 1],c1);patch([0 1 1 1-e 1-e 0+e],[0 0 1 1-e 0+e 0+e],c2);patch([0 0 1 1-e 0+e 0+e],[0 1 1 1-e 1-e 0+e],c3);plot([0 1 1 0 0],[0 0 1 1 0]);disp('+');
  purelin : neural/Transfer Functions/purelin
  "a{2}" : Outport  InitialOutput=[0;0;0;0]
      mask Display: e = 0.06;c1 = [120 230 180]/255;c2 = ([120 230 180]+0)/(256+128);c3 = ([120 230 180]+128)/(256+128);patch([0 1 1 0],[0 0 1 1],c1);patch([0 1 1 1-e 1-e 0+e],[0 0 1 1-e 0+e 0+e],c2);patch([0 0 1 1-e 0+e 0+e],[0 1 1 1-e 1-e 0+e],c3);plot([0 1 1 0 0],[0 0 1 1 0]);
  wires:
  "a{1} "/1 -> Delays 1/1("p{2}")
  Delays 1/1("pd{2,1}") -> "LW{2,1}"/1("ad{2,1}")
  "LW{2,1}"/1("lz{2,1}") -> netsum/1
  "b{2}"/1 -> netsum/2
  netsum/1 -> purelin/1
  purelin/1 -> "a{2}"/1

== system active_with_narx_and_can/NARX Model/NARX Neural Network/Process Input 1 ==
  x : Inport  PortDimensions=21
      mask Display: e = 0.06;c1 = [120 230 180]/255;c2 = ([120 230 180]+0)/(256+128);c3 = ([120 230 180]+128)/(256+128);patch([0 1 1 0],[0 0 1 1],c1);patch([0 1 1 1-e 1-e 0+e],[0 0 1 1-e 0+e 0+e],c2);patch([0 0 1 1-e 0+e 0+e],[0 1 1 1-e 1-e 0+e],c3);plot([0 1 1 0 0],[0 0 1 1 0]);
  mapminmax : neural/Processing Functions/mapminmax  xmin=[-0.0215749510370115069046725864155;-0.118827171696223823915694595144;-0.00235665459206632144431581288302;-0.0190528284886758263183548223196;-0.0035350458990620384734648862235;-0.0338119811284472507328935364512;-0.0241183749752272927335816632421;-0.308457242895283922923255204296;-0.0233904858596965942174605856962;-0.226314075020019406236926329257;-0.024536916029796667498841244992;-0.28605062833296268642868653842;-0.0237761078586202455331655158943;-0.231538449616823988064240325002;-1.01359764284235520648280726164;-0.479982472373988500180530536454;-0.65005336005943559207764792518;-0.0170490280780159833562414917196;-0.00867003225919649525565979786279;-0.00682375693273607093758403863148;-0.0101386611993167542744576081759]  xmax=[0.0258549848429972563279566344363;0.0976182299619778037769179945826;0.00224449140532552698229507015526;0.0141446136733718516587110514138;0.00449695849794220278011769309501;0.0320490629362092660503691377016;0.0279941967057786740558089633168;0.341676473272778724599163524545;0.0267224344963043480838393861632;0.220909367839718900894396824697;0.0275675929617202192245528635794;0.296782256189456306039176070044;0.0275622346339562916683885163138;0.235015433883043356466657769488;1.3245568898335531304866208302;0.403127633225975889885717151628;0.623524263741667139626656535256;0.0176630533929657447533845271437;0.0124610817837135911395618492747;0.00932551090280651570618708490201;0.00836707379926404475056767040542]  ymin=-1  ymax=1
  p : Outport  PortDimensions=21
      mask Display: e = 0.06;c1 = [120 230 180]/255;c2 = ([120 230 180]+0)/(256+128);c3 = ([120 230 180]+128)/(256+128);patch([0 1 1 0],[0 0 1 1],c1);patch([0 1 1 1-e 1-e 0+e],[0 0 1 1-e 0+e 0+e],c2);patch([0 0 1 1-e 0+e 0+e],[0 1 1 1-e 1-e 0+e],c3);plot([0 1 1 0 0],[0 0 1 1 0]);
  wires:
  x/1 -> mapminmax/1
  mapminmax/1 -> p/1

== system active_with_narx_and_can/NARX Model/NARX Neural Network/Process Input 2 ==
  x : Inport  PortDimensions=4
      mask Display: e = 0.06;c1 = [120 230 180]/255;c2 = ([120 230 180]+0)/(256+128);c3 = ([120 230 180]+128)/(256+128);patch([0 1 1 0],[0 0 1 1],c1);patch([0 1 1 1-e 1-e 0+e],[0 0 1 1-e 0+e 0+e],c2);patch([0 0 1 1-e 0+e 0+e],[0 1 1 1-e 1-e 0+e],c3);plot([0 1 1 0 0],[0 0 1 1 0]);
  mapminmax : neural/Processing Functions/mapminmax  xmin=[-1004.30278285339818467036820948;-234.1326937502857958861568477;-867.98317701210100949538173154;-741.850903675889981059299316257]  xmax=[1046.65807806013754088780842721;221.852288007928507340693613514;796.565756640890754169959109277;755.236216304441541069536469877]  ymin=-1  ymax=1
  p : Outport  PortDimensions=4
      mask Display: e = 0.06;c1 = [120 230 180]/255;c2 = ([120 230 180]+0)/(256+128);c3 = ([120 230 180]+128)/(256+128);patch([0 1 1 0],[0 0 1 1],c1);patch([0 1 1 1-e 1-e 0+e],[0 0 1 1-e 0+e 0+e],c2);patch([0 0 1 1-e 0+e 0+e],[0 1 1 1-e 1-e 0+e],c3);plot([0 1 1 0 0],[0 0 1 1 0]);
  wires:
  x/1 -> mapminmax/1
  mapminmax/1 -> p/1

== system active_with_narx_and_can/NARX Model/NARX Neural Network/Process Output 1 ==
  a : Inport  PortDimensions=4
      mask Display: e = 0.06;c1 = [120 230 180]/255;c2 = ([120 230 180]+0)/(256+128);c3 = ([120 230 180]+128)/(256+128);patch([0 1 1 0],[0 0 1 1],c1);patch([0 1 1 1-e 1-e 0+e],[0 0 1 1-e 0+e 0+e],c2);patch([0 0 1 1-e 0+e 0+e],[0 1 1 1-e 1-e 0+e],c3);plot([0 1 1 0 0],[0 0 1 1 0]);
  mapminmax_reverse : neural/Processing Functions/mapminmax_reverse  xmin=[-1004.30278285339818467036820948;-234.1326937502857958861568477;-867.98317701210100949538173154;-741.850903675889981059299316257]  xmax=[1046.65807806013754088780842721;221.852288007928507340693613514;796.565756640890754169959109277;755.236216304441541069536469877]  ymin=-1  ymax=1
  y : Outport  PortDimensions=4
      mask Display: e = 0.06;c1 = [120 230 180]/255;c2 = ([120 230 180]+0)/(256+128);c3 = ([120 230 180]+128)/(256+128);patch([0 1 1 0],[0 0 1 1],c1);patch([0 1 1 1-e 1-e 0+e],[0 0 1 1-e 0+e 0+e],c2);patch([0 0 1 1-e 0+e 0+e],[0 1 1 1-e 1-e 0+e],c3);plot([0 1 1 0 0],[0 0 1 1 0]);
  wires:
  a/1 -> mapminmax_reverse/1
  mapminmax_reverse/1 -> y/1

== system active_with_narx_and_can/NARX Model/NARX Neural Network/Layer 1/Delays 1 ==
  "p{1}" : Inport  PortDimensions=21
      mask Display: e = 0.06;c1 = [120 230 180]/255;c2 = ([120 230 180]+0)/(256+128);c3 = ([120 230 180]+128)/(256+128);patch([0 1 1 0],[0 0 1 1],c1);patch([0 1 1 1-e 1-e 0+e],[0 0 1 1-e 0+e 0+e],c2);patch([0 0 1 1-e 0+e 0+e],[0 1 1 1-e 1-e 0+e],c3);plot([0 1 1 0 0],[0 0 1 1 0]);
  Delay 1 : UnitDelay  InitialCondition=pi_input_1_delayed_1  SampleTime=-1
      mask Display: e = 0.06;c1 = [120 150 230]/255;c2 = ([120 150 230]+0)/383;c3 = ([120 150 230]+128)/383;patch([0 1 1 0],[0 0 1 1],c1);patch([0 1 1 1-e 1-e 0+e],[0 0 1 1-e 0+e 0+e],c2);patch([0 0 1 1-e 0+e 0+e],[0 1 1 1-e 1-e 0+e],c3);plot([0 1 1 0 0],[0 0 1 1 0]);disp('D')
  Delay 2 : UnitDelay  InitialCondition=pi_input_1_delayed_2  SampleTime=-1
      mask Display: e = 0.06;c1 = [120 150 230]/255;c2 = ([120 150 230]+0)/383;c3 = ([120 150 230]+128)/383;patch([0 1 1 0],[0 0 1 1],c1);patch([0 1 1 1-e 1-e 0+e],[0 0 1 1-e 0+e 0+e],c2);patch([0 0 1 1-e 0+e 0+e],[0 1 1 1-e 1-e 0+e],c3);plot([0 1 1 0 0],[0 0 1 1 0]);disp('D')
  mux : Mux  Inputs=2
      mask Display: e = 0.06;c1 = [120 150 230]/255;c2 = ([120 150 230]+0)/383;c3 = ([120 150 230]+128)/383;patch([0 1 1 0],[0 0 1 1],c1);patch([0 1 1 1-e 1-e 0+e],[0 0 1 1-e 0+e 0+e],c2);patch([0 0 1 1-e 0+e 0+e],[0 1 1 1-e 1-e 0+e],c3);plot([0 1 1 0 0],[0 0 1 1 0]);disp('Mux')
  "pd{1,1}" : Outport
      mask Display: e = 0.06;c1 = [120 230 180]/255;c2 = ([120 230 180]+0)/(256+128);c3 = ([120 230 180]+128)/(256+128);patch([0 1 1 0],[0 0 1 1],c1);patch([0 1 1 1-e 1-e 0+e],[0 0 1 1-e 0+e 0+e],c2);patch([0 0 1 1-e 0+e 0+e],[0 1 1 1-e 1-e 0+e],c3);plot([0 1 1 0 0],[0 0 1 1 0]);
  wires:
  "p{1}"/1 -> Delay 1/1
  Delay 1/1 -> Delay 2/1, mux/1
  Delay 2/1 -> mux/2
  mux/1 -> "pd{1,1}"/1

== system active_with_narx_and_can/NARX Model/NARX Neural Network/Layer 1/Delays 2 ==
  "p{1}" : Inport  PortDimensions=4
      mask Display: e = 0.06;c1 = [120 230 180]/255;c2 = ([120 230 180]+0)/(256+128);c3 = ([120 230 180]+128)/(256+128);patch([0 1 1 0],[0 0 1 1],c1);patch([0 1 1 1-e 1-e 0+e],[0 0 1 1-e 0+e 0+e],c2);patch([0 0 1 1-e 0+e 0+e],[0 1 1 1-e 1-e 0+e],c3);plot([0 1 1 0 0],[0 0 1 1 0]);
  Delay 1 : UnitDelay  InitialCondition=pi_input_2_delayed_1  SampleTime=-1
      mask Display: e = 0.06;c1 = [120 150 230]/255;c2 = ([120 150 230]+0)/383;c3 = ([120 150 230]+128)/383;patch([0 1 1 0],[0 0 1 1],c1);patch([0 1 1 1-e 1-e 0+e],[0 0 1 1-e 0+e 0+e],c2);patch([0 0 1 1-e 0+e 0+e],[0 1 1 1-e 1-e 0+e],c3);plot([0 1 1 0 0],[0 0 1 1 0]);disp('D')
  Delay 2 : UnitDelay  InitialCondition=pi_input_2_delayed_2  SampleTime=-1
      mask Display: e = 0.06;c1 = [120 150 230]/255;c2 = ([120 150 230]+0)/383;c3 = ([120 150 230]+128)/383;patch([0 1 1 0],[0 0 1 1],c1);patch([0 1 1 1-e 1-e 0+e],[0 0 1 1-e 0+e 0+e],c2);patch([0 0 1 1-e 0+e 0+e],[0 1 1 1-e 1-e 0+e],c3);plot([0 1 1 0 0],[0 0 1 1 0]);disp('D')
  mux : Mux  Inputs=2
      mask Display: e = 0.06;c1 = [120 150 230]/255;c2 = ([120 150 230]+0)/383;c3 = ([120 150 230]+128)/383;patch([0 1 1 0],[0 0 1 1],c1);patch([0 1 1 1-e 1-e 0+e],[0 0 1 1-e 0+e 0+e],c2);patch([0 0 1 1-e 0+e 0+e],[0 1 1 1-e 1-e 0+e],c3);plot([0 1 1 0 0],[0 0 1 1 0]);disp('Mux')
  "pd{1,2}" : Outport
      mask Display: e = 0.06;c1 = [120 230 180]/255;c2 = ([120 230 180]+0)/(256+128);c3 = ([120 230 180]+128)/(256+128);patch([0 1 1 0],[0 0 1 1],c1);patch([0 1 1 1-e 1-e 0+e],[0 0 1 1-e 0+e 0+e],c2);patch([0 0 1 1-e 0+e 0+e],[0 1 1 1-e 1-e 0+e],c3);plot([0 1 1 0 0],[0 0 1 1 0]);
  wires:
  "p{1}"/1 -> Delay 1/1
  Delay 1/1 -> Delay 2/1, mux/1
  Delay 2/1 -> mux/2
  mux/1 -> "pd{1,2}"/1
